simulink model "experiments_actuate_pendulum_orderly"  (Simulink 7.8)
settings: Solver=ode1  StartTime=0.0  StopTime=inf  FixedStep=0.001  RelTol=1e-3
PreLoadFcn:
  | init_pnp_control
InitFcn:
  | init_pnp_control
values from neighbouring files (symbols this model uses):
  g = [0 0 -9.81]'    [control_initfcn.m]
undefined symbols (not defined in the file or in its folder): a0, ampl_wn, b0, baseOffset_x, baseOffset_y, baseOffset_z, cobotNa, K, l, m, magnitude, omega, omega_n, phase_wn, pose, T, TA, zeta
libraries: simulink x1, rtai_utilities x1
settings Model: Creator=mkarmann  LastModifiedBy=mkarmann  SimulationMode=external
settings DataIOCC: LimitDataPoints=off
settings RTWCC: SystemTargetFile=prt.tlc  TemplateMakefile=prt.tmf  Description=Linux PREEMPT_RT Real-Time Target  ProcessScript=prt_make_rtw_hook
settings STFCustomTargetCC: TargetFunctionLibrary=GNU99 (GNU)  ModelReferenceCompliant=off  SystemTargetFile=prt.tlc
settings GRTTargetCC: TargetFunctionLibrary=GNU99 (GNU)  ModelReferenceCompliant=off  ParMdlRefBuildCompliant=off  CompOptLevelCompliant=off  ConcurrentExecutionCompliant=off  MatFileLogging=off  ExtMode=on  ExtModeMexArgs=cobotNb

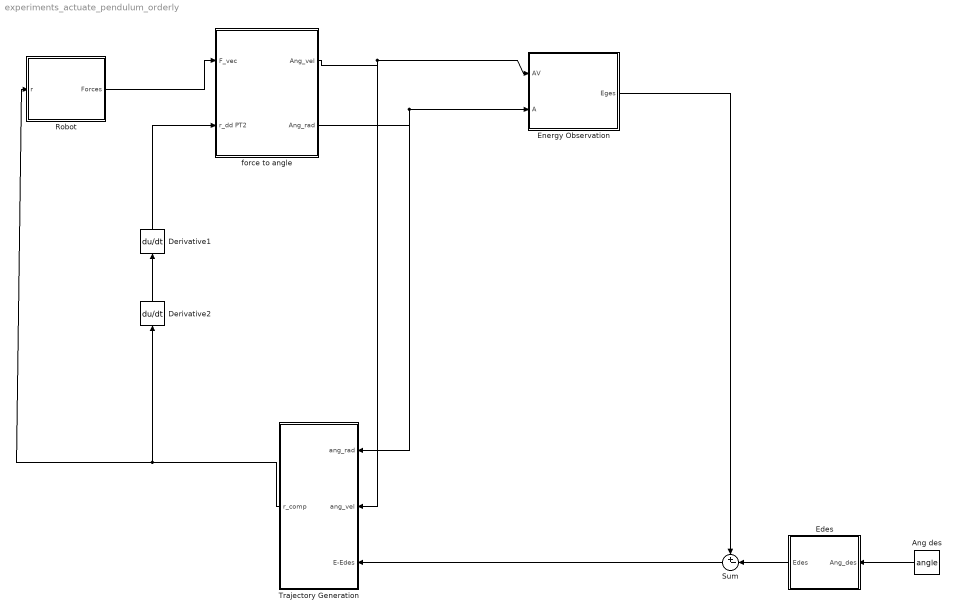
== system experiments_actuate_pendulum_orderly ==
  Ang des : Constant  Value=angle
  Derivative1 : Derivative
  Derivative2 : Derivative
  Edes : Subsystem
  Energy Observation : Subsystem
  Robot : Subsystem
  Sum : Sum  Inputs=+-|
  Trajectory Generation : Subsystem
  force to angle : Subsystem
  wires:
  Energy Observation/1(Eges) -> Sum/1
  Ang des/1 -> Edes/1(Ang_des)
  Edes/1(Edes) -> Sum/2
  Trajectory Generation/1(r_comp) -> Robot/1(r), Derivative2/1
  Robot/1(Forces) -> force to angle/1(F_vec)
  Sum/1 -> Trajectory Generation/3(E-Edes)
  force to angle/2(Ang_rad) -> Energy Observation/2(A), Trajectory Generation/1(ang_rad)
  force to angle/1(Ang_vel) -> Energy Observation/1(AV), Trajectory Generation/2(ang_vel)
  Derivative2/1 -> Derivative1/1
  Derivative1/1 -> force to angle/2(r_dd PT2)

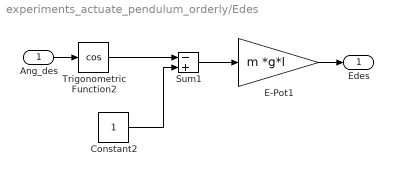
== system experiments_actuate_pendulum_orderly/Edes ==
  Ang_des : Inport
  Constant2 : Constant
  E-Pot1 : Gain  Gain=m *g*l
  Sum1 : Sum  Inputs=-|+
  Trigonometric Function2 : Trigonometry  Operator=cos
  Edes : Outport
  wires:
  E-Pot1/1 -> Edes/1
  Ang_des/1 -> Trigonometric Function2/1
  Sum1/1 -> E-Pot1/1
  Constant2/1 -> Sum1/2
  Trigonometric Function2/1 -> Sum1/1

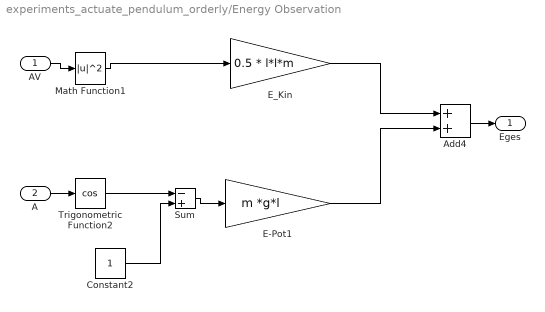
== system experiments_actuate_pendulum_orderly/Energy Observation ==
  AV : Inport
  A : Inport  Port=2
  Add4 : Sum
  Constant2 : Constant
  E-Pot1 : Gain  Gain=m *g*l
  E_Kin : Gain  Gain=0.5 * l*l*m
  Math Function1 : Math  Operator=magnitude^2  SaturateOnIntegerOverflow=on
  Sum : Sum  Inputs=-|+
  Trigonometric Function2 : Trigonometry  Operator=cos
  Eges : Outport
  wires:
  Math Function1/1 -> E_Kin/1
  Sum/1 -> E-Pot1/1
  Constant2/1 -> Sum/2
  Trigonometric Function2/1 -> Sum/1
  E_Kin/1 -> Add4/1
  E-Pot1/1 -> Add4/2
  AV/1 -> Math Function1/1
  Add4/1 -> Eges/1
  A/1 -> Trigonometric Function2/1

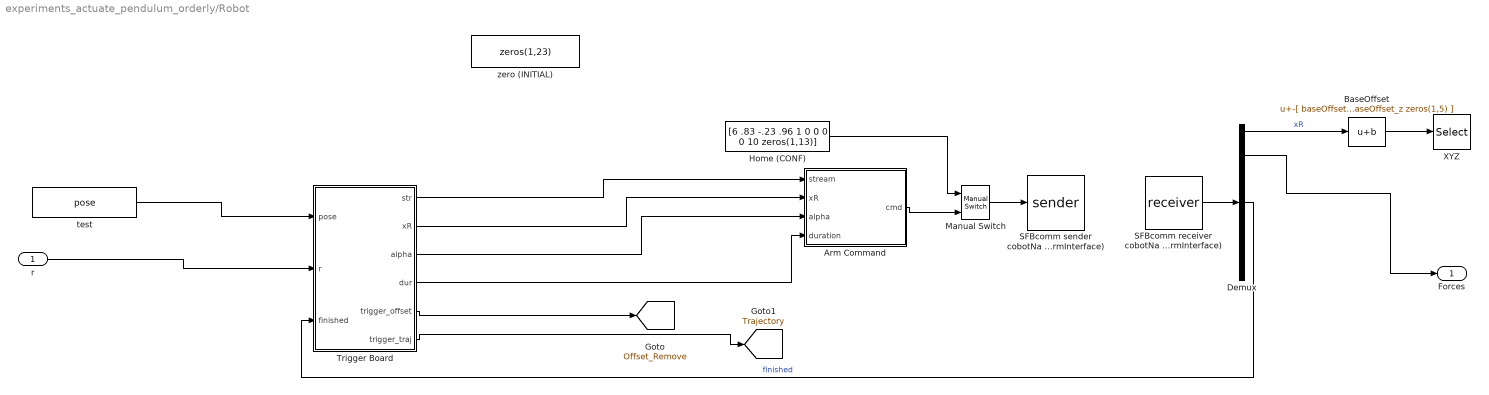
== system experiments_actuate_pendulum_orderly/Robot ==
  r : Inport
  Arm Command : Subsystem
  BaseOffset : Bias  Bias="-[ baseOffset_x  baseOffset_y  baseOffset_z zeros(1,5) ]"
  Demux : Demux  Outputs=[8 6 7 1 1 1 1]
  Home (CONF) : Constant  Value=[6 .83 -.23 .96 1 0 0 0 0 10 zeros(1,13)]  SampleTime=TA
  Manual Switch : simulink/Signal Routing/Manual Switch  sw=0  action=0  varsize=off
  SFBcomm receiver cobotNa (ArmInterface) : S-Function  AncestorBlock=sfbc_lib/SFBcomm receiver  FunctionName=receiver  Parameters=localPort streamID remoteSettings portNames portWidths sampleTime outputLatency outputIdleTime connectTimeout  EnableBusSupport=off  mask(SFBcomm){localPort=8666, streamID=3, remoteSettings=[cobotNa ':8665'], portNames=A, portWidths=25, outputLatency=off, outputIdleTime=off, connectTimeout=200, sampleTime=TA}
      mask prompts: localPort "Local Port"; streamID "Stream ID"; remoteSettings "Remote Settings"; portNames "Port Names"; portWidths "Port Widths"; outputLatency "Output Latency"; outputIdleTime "Output Idle Time"; connectTimeout "Connect Timeout (in ms)"; sampleTime "Sample Time (-1 for inherited):"
      mask help: Receives data via SFB comm
      mask init:
      | idx=[0 strfind(portNames,' ') length(portNames)];
      | ddt=strfind(outputLatency,'on');
      | dit=strfind(outputIdleTime,'on');
      | 
      | for i=1:17
      |  if(i<length(idx))
      |   portnumber(i)=i;
      |   label{i}=portNames(idx(i)+1:idx(i+1));
      |  elseif((i==length(idx))&&(length(ddt)>0))
      |   portnumber(i)=i;
      |   label{i}='dt';
      |  elseif((i==length(idx))&&(length(dit)>0))
      |   portnumber(i)=i;
      |   label{i}='it';
      |  elseif((i==length(idx)+1)&&(length(ddt)>0)&&(length(dit)>0))
      |   portnumber(i)=i;
      |   label{i}='it';
      |  else
      |   portnumber(i)=1;
      |   label{i}=label{1};
      |  end
      | end
      mask Display:
      | image(imread('sfbcomm1.bmp'))
      | 
      | port_label('output',portnumber( 1),label{ 1})
      | port_label('output',portnumber( 2),label{ 2})
      | port_label('output',portnumber( 3),label{ 3})
      | port_label('output',portnumber( 4),label{ 4})
      | port_label('output',portnumber( 5),label{ 5})
      | port_label('output',portnumber( 6),label{ 6})
      | port_label('output',portnumber( 7),label{ 7})
      | port_label('output',portnumber( 8),label{ 8})
      | port_label('output',portnumber( 9),label{ 9})
      | port_label('output',portnumber(10),label{10})
      | port_label('output',portnumber(11),label{11})
      | port_label('output',portnumber(12),label{12})
      | port_label('output',portnumber(13),label{13})
      | port_label('output',portnumber(14),label{14})
      | port_label('output',portnumber(15),label{15})
      | port_label('output',portnumber(16),label{16})
      | port_label('output',portnumber(17),label{17})
  SFBcomm sender cobotNa (ArmInterface) : S-Function  AncestorBlock=sfbc_lib/SFBcomm sender  FunctionName=sender  Parameters=localPort streamID remoteSettings portNames sampleTime connectTimeout  EnableBusSupport=off  mask(SFBcomm){localPort=8566, streamID=2, remoteSettings=[cobotNa ':8565'], portNames=A, connectTimeout=200, sampleTime=-1}
      mask prompts: localPort "Local Port"; streamID "Stream ID"; remoteSettings "Remote Settings"; portNames "Port Names"; connectTimeout "Connect Timeout (in ms)"; sampleTime "Sample time (-1 for inherited):"
      mask help: Sends data via SFB comm
      mask init:
      | idx=[0 strfind(portNames,' ') length(portNames)];
      | 
      | for i=1:16
      |  if(i<length(idx))
      |   portnumber(i)=i;
      |   label{i}=portNames(idx(i)+1:idx(i+1));
      |  else
      |   portnumber(i)=1;
      |   label{i}=label{1};
      |  end
      | end
      mask Display:
      | image(imread('sfbcomm1.bmp'))
      | port_label('input',portnumber( 1),label{ 1})
      | port_label('input',portnumber( 2),label{ 2})
      | port_label('input',portnumber( 3),label{ 3})
      | port_label('input',portnumber( 4),label{ 4})
      | port_label('input',portnumber( 5),label{ 5})
      | port_label('input',portnumber( 6),label{ 6})
      | port_label('input',portnumber( 7),label{ 7})
      | port_label('input',portnumber( 8),label{ 8})
      | port_label('input',portnumber( 9),label{ 9})
      | port_label('input',portnumber(10),label{10})
      | port_label('input',portnumber(11),label{11})
      | port_label('input',portnumber(12),label{12})
      | port_label('input',portnumber(13),label{13})
      | port_label('input',portnumber(14),label{14})
      | port_label('input',portnumber(15),label{15})
      | port_label('input',portnumber(16),label{16})
  Trigger Board : MATLAB Function  TreatAsAtomicUnit=on
  XYZ : Selector  InputPortWidth=8  IndexOptions=Index vector (dialog)  Indices=[1:3]  OutputSizes=1
  test : Constant  Value=pose  SampleTime=TA
  zero (INITIAL) : Constant  Value=zeros(1,23)  SampleTime=TA
  Forces : Outport
  tag scope: Offset_Remove=global, Trajectory=global
  wires:
  test/1 -> Trigger Board/1(pose)
  SFBcomm receiver cobotNa (ArmInterface)/1 -> Demux/1
  Demux/1 -> BaseOffset/1  "xR"
  Manual Switch/1 -> SFBcomm sender cobotNa (ArmInterface)/1
  Arm Command/1(cmd) -> Manual Switch/2
  BaseOffset/1 -> XYZ/1
  Demux/2 -> Forces/1
  Trigger Board/3(alpha) -> Arm Command/3(alpha)
  Trigger Board/2(xR) -> Arm Command/2(xR)
  Home (CONF)/1 -> Manual Switch/1
  Trigger Board/4(dur) -> Arm Command/4(duration)
  Trigger Board/5(trigger_offset) -> [Offset_Remove]
  Trigger Board/6(trigger_traj) -> [Trajectory]
  r/1 -> Trigger Board/2(r)
  Trigger Board/1(str) -> Arm Command/1(stream)
  Demux/4 -> Trigger Board/3(finished)  "finished"

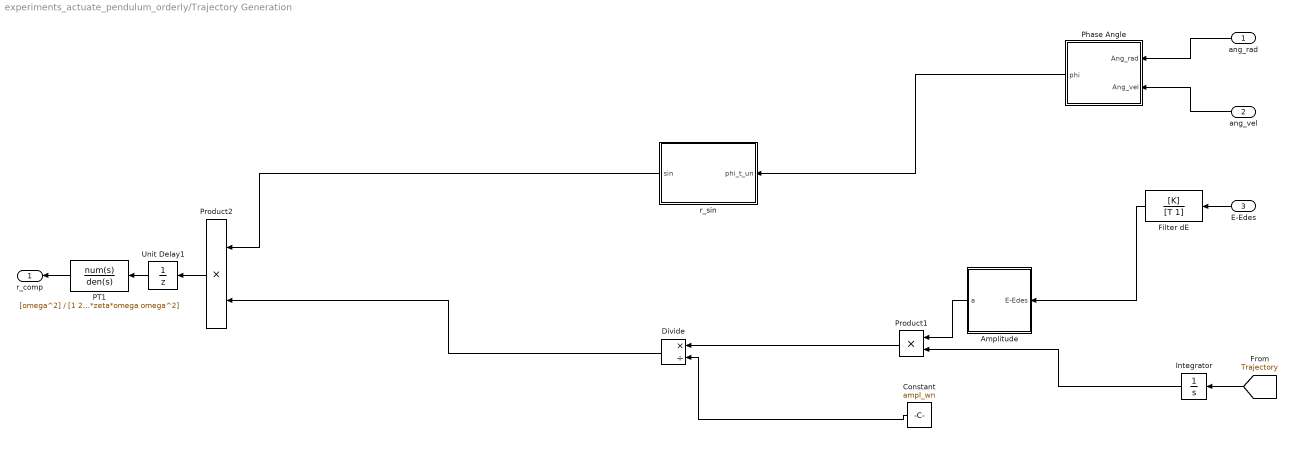
== system experiments_actuate_pendulum_orderly/Trajectory Generation ==
  ang_rad : Inport
  ang_vel : Inport  Port=2
  E-Edes : Inport  Port=3
  Amplitude : Subsystem
  Constant : Constant  Value=ampl_wn
  Divide : Product  Inputs=*/
  Filter dE : TransferFcn  Numerator=[K]  Denominator=[T 1]
  Integrator : Integrator  LimitOutput=on  UpperSaturationLimit=1  LowerSaturationLimit=0
  PT1 : TransferFcn  Numerator=[omega^2]  Denominator=[1 2*zeta*omega omega^2]
  Phase Angle : Subsystem
  Product1 : Product  Inputs=**
  Product2 : Product  RndMeth=Zero
  Unit Delay1 : UnitDelay  SampleTime=-1
  r_sin : Subsystem
  r_comp : Outport
  wires:
  Unit Delay1/1 -> PT1/1
  Product2/1 -> Unit Delay1/1
  [Trajectory] -> Integrator/1
  Constant/1 -> Divide/2
  E-Edes/1 -> Filter dE/1
  Amplitude/1(a) -> Product1/1
  Integrator/1 -> Product1/2
  ang_rad/1 -> Phase Angle/1(Ang_rad)
  ang_vel/1 -> Phase Angle/2(Ang_vel)
  Product1/1 -> Divide/1
  r_sin/1(sin) -> Product2/1
  Divide/1 -> Product2/2
  Filter dE/1 -> Amplitude/1(E-Edes)
  PT1/1 -> r_comp/1
  Phase Angle/1(phi) -> r_sin/1(phi_t_un)

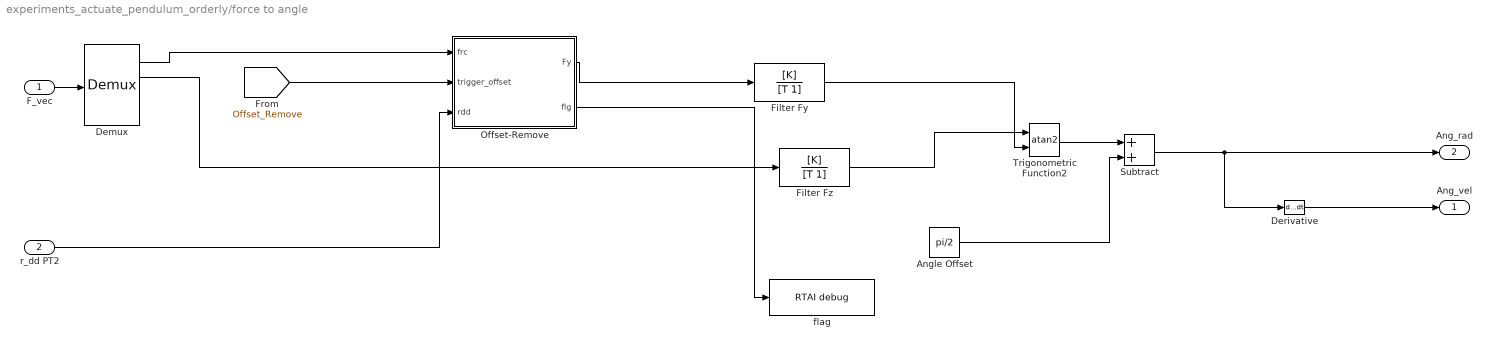
== system experiments_actuate_pendulum_orderly/force to angle ==
  F_vec : Inport
  r_dd PT2 : Inport  Port=2
  Angle Offset : Constant  Value=pi/2
  Demux : Demux  Outputs=6
  Derivative : Derivative
  Filter Fy : TransferFcn  Numerator=[K]  Denominator=[T 1]
  Filter Fz : TransferFcn  Numerator=[K]  Denominator=[T 1]
  Offset-Remove : MATLAB Function  TreatAsAtomicUnit=on
  Subtract : Sum
  Trigonometric Function2 : Trigonometry  Operator=atan2
  flag : rtai_utilities/RTAI debug  rate=10
  Ang_vel : Outport
  Ang_rad : Outport  Port=2
  wires:
  F_vec/1 -> Demux/1
  Demux/3 -> Filter Fz/1
  Demux/2 -> Offset-Remove/1(frc)
  [Offset_Remove] -> Offset-Remove/2(trigger_offset)
  Offset-Remove/1(Fy) -> Filter Fy/1
  Filter Fz/1 -> Trigonometric Function2/1
  Filter Fy/1 -> Trigonometric Function2/2
  Trigonometric Function2/1 -> Subtract/1
  Angle Offset/1 -> Subtract/2
  Subtract/1 -> Ang_rad/1, Derivative/1
  Derivative/1 -> Ang_vel/1
  Offset-Remove/2(flg) -> flag/1
  r_dd PT2/1 -> Offset-Remove/3(rdd)

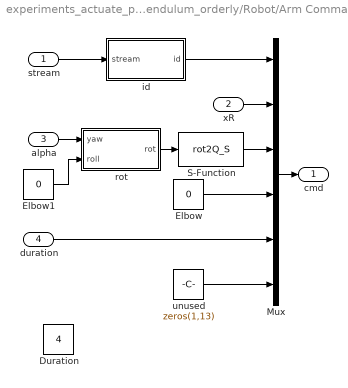
== system experiments_actuate_pendulum_orderly/Robot/Arm Command ==
  stream : Inport
  xR : Inport  Port=2
  alpha : Inport  Port=3
  duration : Inport  Port=4
  Duration : Constant  Value=4
  Elbow : Constant  Value=0
  Elbow1 : Constant  Value=0
  Mux : Mux  Inputs=[1 3 4 1 1 13]
  S-Function : S-Function  FunctionName=rot2Q_S  EnableBusSupport=off
  id : MATLAB Function  TreatAsAtomicUnit=on
  rot : MATLAB Function  TreatAsAtomicUnit=on
  unused : Constant  Value=zeros(1,13)
  cmd : Outport
  wires:
  rot/1(rot) -> S-Function/1
  Elbow/1 -> Mux/4
  S-Function/1 -> Mux/3
  Elbow1/1 -> rot/2(roll)
  xR/1 -> Mux/2
  alpha/1 -> rot/1(yaw)
  Mux/1 -> cmd/1
  stream/1 -> id/1(stream)
  id/1(id) -> Mux/1
  unused/1 -> Mux/6
  duration/1 -> Mux/5

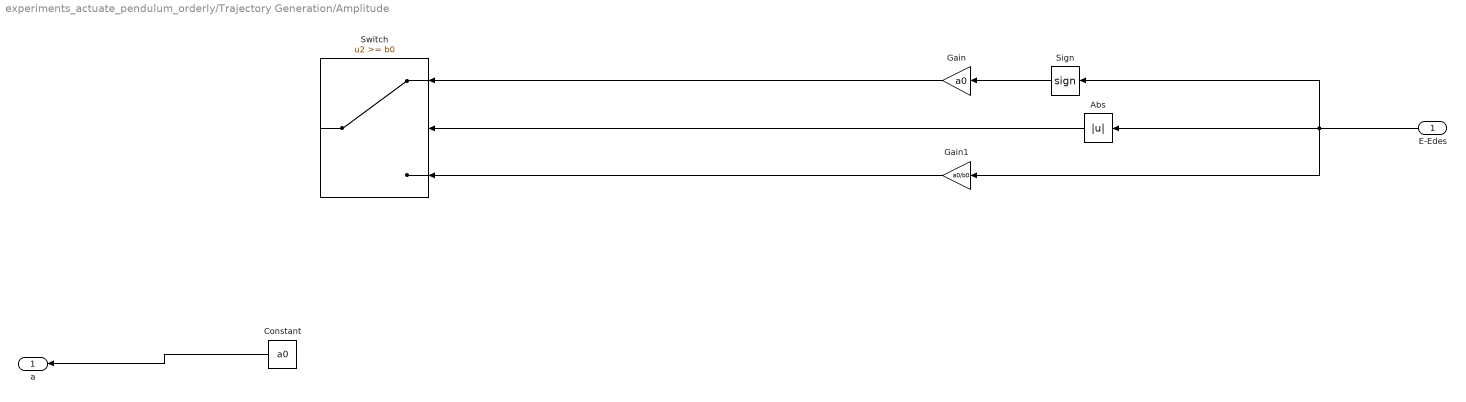
== system experiments_actuate_pendulum_orderly/Trajectory Generation/Amplitude ==
  E-Edes : Inport
  Abs : Abs
  Constant : Constant  Value=a0
  Gain : Gain  Gain=a0
  Gain1 : Gain  Gain=a0/b0
  Sign : Signum
  Switch : Switch  Threshold=b0
  a : Outport
  wires:
  Gain1/1 -> Switch/3
  Gain/1 -> Switch/1
  Sign/1 -> Gain/1
  Abs/1 -> Switch/2
  E-Edes/1 -> Abs/1, Sign/1, Gain1/1
  Constant/1 -> a/1

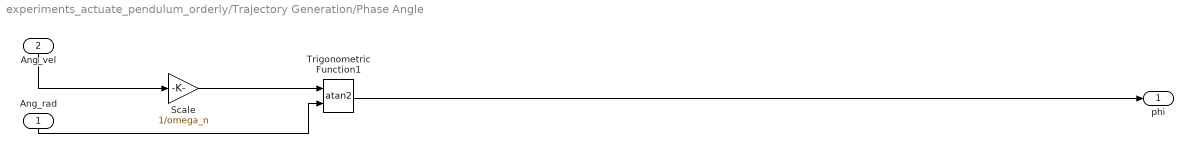
== system experiments_actuate_pendulum_orderly/Trajectory Generation/Phase Angle ==
  Ang_rad : Inport
  Ang_vel : Inport  Port=2
  Scale : Gain  Gain=1/omega_n
  Trigonometric Function1 : Trigonometry  Operator=atan2
  phi : Outport
  wires:
  Trigonometric Function1/1 -> phi/1
  Ang_vel/1 -> Scale/1
  Ang_rad/1 -> Trigonometric Function1/2
  Scale/1 -> Trigonometric Function1/1

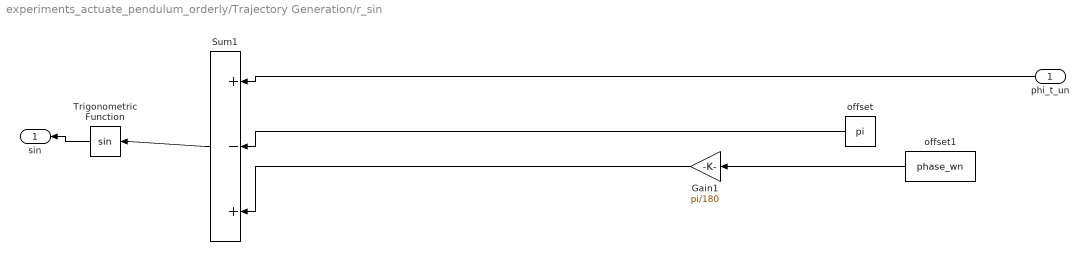
== system experiments_actuate_pendulum_orderly/Trajectory Generation/r_sin ==
  phi_t_un : Inport
  Gain1 : Gain  Gain=pi/180
  Sum1 : Sum  Inputs=+|-|+
  Trigonometric Function : Trigonometry
  offset : Constant  Value=pi
  offset1 : Constant  Value=phase_wn
  sin : Outport
  wires:
  offset1/1 -> Gain1/1
  Sum1/1 -> Trigonometric Function/1
  offset/1 -> Sum1/2
  phi_t_un/1 -> Sum1/1
  Trigonometric Function/1 -> sin/1
  Gain1/1 -> Sum1/3

== matlab function Robot/Arm Command/id ==
  data: stream input double; id output double
function id = fcn(stream)
%#eml

if stream == 1
    id = 29;
else
    id = 6;
end

end

== matlab function Robot/Arm Command/rot ==
  data: yaw input double; rot output double; roll input double
function rot = fcn(yaw,roll)
%#eml

rotZ = [ cos(yaw)  -sin(yaw) 0;
         sin(yaw)  cos(yaw)  0;
          0          0       1 ];
    
rotX = [ 1       0       0;
        0   cos(roll) -sin(roll);
        0   sin(roll)  cos(roll) ];
    
rot = rotZ * rotX;

== matlab function force to angle/Offset-Remove ==
  data: frc input double; Fy output double; trigger_offset input double; rdd input double; M_EE parameter double; flg output double
function [Fy, flg] = fcn(frc, trigger_offset, rdd, M_EE)
%#codegen

persistent cnt;
persistent force;
persistent av;
persistent flag;

if(isempty(cnt))
     cnt = 0;
     force = 0;
     av = 0;
     flag = 0;
end

if(trigger_offset == 1)
    cnt = cnt + 1;

    if(cnt < 4002)
        force = force + frc;
        av = force;
        flag = 0;
    elseif(cnt == 4002)
        av = force/cnt;
        flag = 1;
    end
    
    if (flag == 1)
        Fy = frc - av+ rdd*M_EE*1.1;
    else
        Fy = frc;
    end
    
else
    Fy = frc;
    
end

flg = av;

end

== matlab function Robot/Trigger Board ==
  data: pose input double; str output double; r input double; finished input double; xR output double; alpha output double; dur output double; trigger_offset output double; trigger_traj output double
function [str, xR, alpha, dur, trigger_offset, trigger_traj] = fcn(pose, r, finished)
%#codegen

% init

persistent wait;
persistent step;                            % Step = 0 => feed pose, step = 1 => feed stream
persistent stream;                          % position or feed
persistent vector;                          % content
persistent duration;
persistent cnt;
persistent to;                              % trigger_offset
persistent tt;                              % trigger_traj



if(isempty(wait))
    wait = 0;
    cnt = 0;
    duration = 4;
    to = 0;
    tt = 0;
    step = 0;
    stream = 0;
    vector = [0 0 0 0 0];
end

% Time Parameter

cnt = cnt + 1;



switch step
    
    case 0
            stream = 0;
            vector = pose;
            duration = 4;
            
            if(cnt >= 6000 && finished == 1)
                to = 1;
            end 
            
            if(cnt >= 11000)
                step = 1;
            end
    case 1
            stream = 0;
            vector = [pose(1), 0.05+pose(2) , pose(3), 0];
            duration = 0.5;
            
            if(cnt >= 20000 && finished == 1)
                step = 2;
                tt = 1;
            end
            
    case 2
            stream = 1;
            vector = [pose(1), r+0.05+pose(2) , pose(3), 0];
            
           
end



% output

str = stream;
xR = [vector(1), vector(2), vector(3)];
alpha = vector(4);
dur = duration;
trigger_offset = to;
trigger_traj = tt;

end
